simulink model "PDQuadrotor"  (Simulink 7.7)
settings: Solver=ode4  StartTime=0.0  StopTime=10.0  FixedStep=0.2  RelTol=1e-3
values from neighbouring files (symbols this model uses):
  b = 3.13*10^(-5)    (= 3.13e-05)    [Quadparameters.m]
  d = 7.5*10^(-7)    (= 7.5e-07)    [Quadparameters.m]
  g = 9.81    [Quadparameters.m]
  Ix = 7.5*10^(-3)    (= 0.0075)    [Quadparameters.m]
  Iy = 7.5*10^(-3)    (= 0.0075)    [Quadparameters.m]
  Iz = 1.3*10^(-2)    (= 0.013)    [Quadparameters.m]
  Jr = 6.5*10^(-5)    (= 6.5e-05)    [Quadparameters.m]
  kdp = 0.4    [Quadparameters.m]
  kdps = 0.4    [Quadparameters.m]
  kdt = 0.4    [Quadparameters.m]
  kdz = 20    [Quadparameters.m]
  kpp = 0.8    [Quadparameters.m]
  kpps = 1    [Quadparameters.m]
  kpt = 1.2    [Quadparameters.m]
  kpz = 100    [Quadparameters.m]
  l = 0.23    [Quadparameters.m]
  m = 0.65    [Quadparameters.m]
libraries: simulink x2
settings Model: Creator=abdelrazzak.merheb  LastModifiedBy=ISIT-Eric J.Huang
settings DebuggingCC: StrictBusMsg=Warning

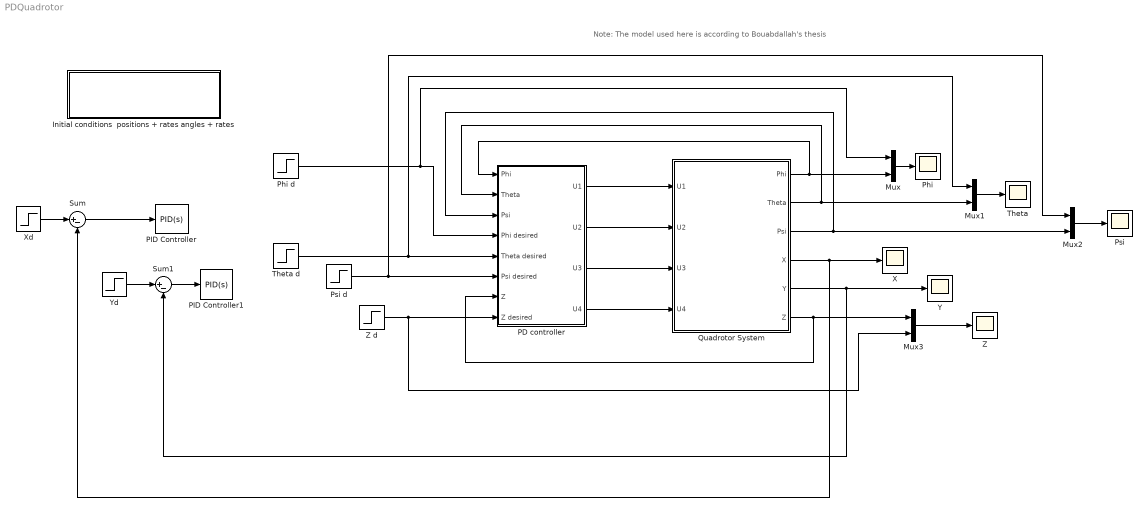
== system PDQuadrotor ==
  note: Note:
      | The model used here is according to Bouabdallah's thesis
  Initial conditions  positions + rates angles + rates : Subsystem  mask{x0=0, y0=0, z0=1, x0dot=0, y0dot=0, z0dot=0, phi0=0, theta0=0, psi0=0, phi0dot=0, theta0dot=0, psi0dot=0}
      mask prompts: x0 "Initial X position, in meters"; y0 "Initial Y position, in meters"; z0 "Initial Z position, in meters"; x0dot "Initial Velocity in X direction, m/sec"; y0dot "Initial Velocity in Y direction, m/sec"; z0dot "Initial Velocity in Z direction, m/sec"; phi0 "Initial Roll angle, deg"; theta0 "Initial Pitch angle, deg"; psi0 "Initial Yaw angle, deg"; phi0dot "Initial Roll rate, deg/sec"; theta0dot "Initial Pitch rate, deg/sec"; psi0dot "Initial Yaw rate, deg/sec"
      mask Display: disp('Enter initial conditions here')
  Mux{,1..3} (4 alike) : Mux  Inputs=2
  PD controller : Subsystem
  PID Controller : simulink/Continuous/PID Controller  SystemSampleTime=-1  Controller=PID  TimeDomain=Continuous-time  SampleTime=1  IntegratorMethod=Forward Euler  FilterMethod=Forward Euler  Form=Parallel  P=1  I=0  D=0  N=100  InitialConditionSource=internal  InitialConditionForIntegrator=0  InitialConditionForFilter=0  ExternalReset=none  LimitOutput=off  UpperSaturationLimit=inf  LowerSaturationLimit=-inf  LinearizeAsGain=off  AntiWindupMode=none  Kb=1  TrackingMode=off  Kt=1  PParamMin=[]  PParamMax=[]  IParamMin=[]  IParamMax=[]  DParamMin=[]  DParamMax=[]  NParamMin=[]  NParamMax=[]  KbParamMin=[]  KbParamMax=[]  KtParamMin=[]  KtParamMax=[]  POutMin=[]  POutMax=[]  IOutMin=[]  IOutMax=[]  DOutMin=[]  DOutMax=[]  NOutMin=[]  NOutMax=[]  KbOutMin=[]  KbOutMax=[]  KtOutMin=[]  KtOutMax=[]  IntegratorOutMin=[]  IntegratorOutMax=[]  FilterOutMin=[]  FilterOutMax=[]  SumOutMin=[]  SumOutMax=[]  SumI1OutMin=[]  SumI1OutMax=[]  SumI2OutMin=[]  SumI2OutMax=[]  SumI3OutMin=[]  SumI3OutMax=[]  SumDOutMin=[]  SumDOutMax=[]  SaturationOutMin=[]  SaturationOutMax=[]  IntegratorContinuousStateAttributes=''  IntegratorStateMustResolveToSignalObject=off  IntegratorRTWStateStorageClass=Auto  FilterContinuousStateAttributes=''  FilterStateMustResolveToSignalObject=off  FilterRTWStateStorageClass=Auto
  PID Controller1 : simulink/Continuous/PID Controller  SystemSampleTime=-1  Controller=PID  TimeDomain=Continuous-time  SampleTime=1  IntegratorMethod=Forward Euler  FilterMethod=Forward Euler  Form=Parallel  P=1  I=0  D=0  N=100  InitialConditionSource=internal  InitialConditionForIntegrator=0  InitialConditionForFilter=0  ExternalReset=none  LimitOutput=off  UpperSaturationLimit=inf  LowerSaturationLimit=-inf  LinearizeAsGain=off  AntiWindupMode=none  Kb=1  TrackingMode=off  Kt=1  PParamMin=[]  PParamMax=[]  IParamMin=[]  IParamMax=[]  DParamMin=[]  DParamMax=[]  NParamMin=[]  NParamMax=[]  KbParamMin=[]  KbParamMax=[]  KtParamMin=[]  KtParamMax=[]  POutMin=[]  POutMax=[]  IOutMin=[]  IOutMax=[]  DOutMin=[]  DOutMax=[]  NOutMin=[]  NOutMax=[]  KbOutMin=[]  KbOutMax=[]  KtOutMin=[]  KtOutMax=[]  IntegratorOutMin=[]  IntegratorOutMax=[]  FilterOutMin=[]  FilterOutMax=[]  SumOutMin=[]  SumOutMax=[]  SumI1OutMin=[]  SumI1OutMax=[]  SumI2OutMin=[]  SumI2OutMax=[]  SumI3OutMin=[]  SumI3OutMax=[]  SumDOutMin=[]  SumDOutMax=[]  SaturationOutMin=[]  SaturationOutMax=[]  IntegratorContinuousStateAttributes=''  IntegratorStateMustResolveToSignalObject=off  IntegratorRTWStateStorageClass=Auto  FilterContinuousStateAttributes=''  FilterStateMustResolveToSignalObject=off  FilterRTWStateStorageClass=Auto
  Phi : Scope
  Phi d : Step  After=0  SampleTime=0
  Psi : Scope
      settings: SaveName=ScopeData2
  Psi d : Step  After=0  SampleTime=0
  Quadrotor System : Subsystem
  Sum : Sum  Inputs=|+-
  Sum1 : Sum  Inputs=|+-
  Theta : Scope
  Theta d : Step  After=0.5  SampleTime=0
  X : Scope
      settings: SaveName=ScopeData3
  Xd : Step  Time=3  After=40  SampleTime=0
  Y : Scope
      settings: SaveName=ScopeData5
  Yd : Step  Time=5  After=35  SampleTime=0
  Z : Scope
      settings: SaveName=ScopeData4
  Z d : Step  Time=0  After=10  SampleTime=0
  wires:
  PD controller/1(U1) -> Quadrotor System/1(U1)
  PD controller/2(U2) -> Quadrotor System/2(U2)
  PD controller/3(U3) -> Quadrotor System/3(U3)
  PD controller/4(U4) -> Quadrotor System/4(U4)
  Quadrotor System/6(Z) -> PD controller/7(Z), Mux3/1
  Quadrotor System/1(Phi) -> PD controller/1(Phi), Mux/2
  Quadrotor System/2(Theta) -> PD controller/2(Theta), Mux1/2
  Quadrotor System/3(Psi) -> PD controller/3(Psi), Mux2/2
  Psi d/1 -> PD controller/6(Psi desired), Mux2/1
  Z d/1 -> PD controller/8(Z desired), Mux3/2
  Quadrotor System/5(Y) -> Y/1, Sum1/2
  Quadrotor System/4(X) -> X/1, Sum/2
  Mux/1 -> Phi/1
  Mux1/1 -> Theta/1
  Mux2/1 -> Psi/1
  Mux3/1 -> Z/1
  Sum1/1 -> PID Controller1/1
  Xd/1 -> Sum/1
  Sum/1 -> PID Controller/1
  Yd/1 -> Sum1/1
  Phi d/1 -> PD controller/4(Phi desired), Mux/1
  Theta d/1 -> PD controller/5(Theta desired), Mux1/1

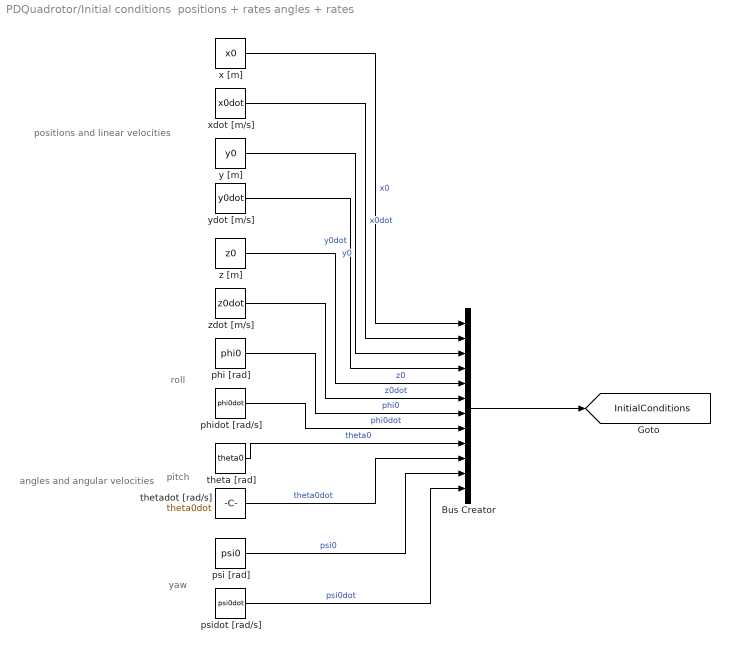
== system PDQuadrotor/Initial conditions  positions + rates angles + rates ==
  note: positions and linear velocities
  note: angles and angular velocities
  note: yaw
  note: pitch
  note: roll
  Bus Creator : BusCreator  Inputs=12
  phi [rad] : Constant  Value=phi0
  phidot [rad/s] : Constant  Value=phi0dot
  psi [rad] : Constant  Value=psi0
  psidot [rad/s] : Constant  Value=psi0dot
  theta [rad] : Constant  Value=theta0
  thetadot [rad/s] : Constant  Value=theta0dot
  x [m] : Constant  Value=x0
  xdot [m/s] : Constant  Value=x0dot
  y [m] : Constant  Value=y0
  ydot [m/s] : Constant  Value=y0dot
  z [m] : Constant  Value=z0
  zdot [m/s] : Constant  Value=z0dot
  tag scope: InitialConditions=global
  wires:
  x [m]/1 -> Bus Creator/1  "x0"
  xdot [m/s]/1 -> Bus Creator/2  "x0dot"
  y [m]/1 -> Bus Creator/3  "y0"
  ydot [m/s]/1 -> Bus Creator/4  "y0dot"
  z [m]/1 -> Bus Creator/5  "z0"
  zdot [m/s]/1 -> Bus Creator/6  "z0dot"
  phi [rad]/1 -> Bus Creator/7  "phi0"
  phidot [rad/s]/1 -> Bus Creator/8  "phi0dot"
  theta [rad]/1 -> Bus Creator/9  "theta0"
  thetadot [rad/s]/1 -> Bus Creator/10  "theta0dot"
  psi [rad]/1 -> Bus Creator/11  "psi0"
  psidot [rad/s]/1 -> Bus Creator/12  "psi0dot"
  Bus Creator/1 -> [InitialConditions]

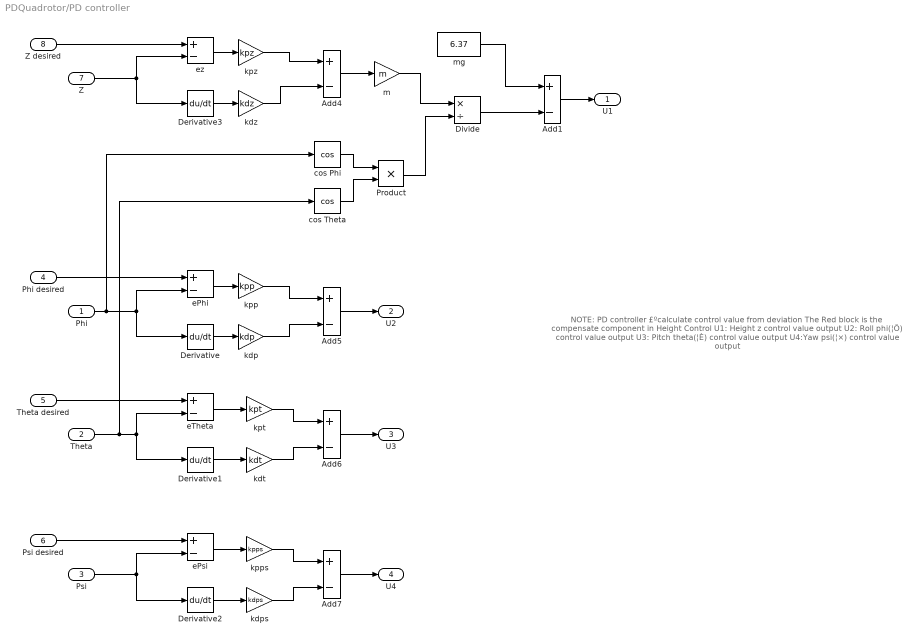
== system PDQuadrotor/PD controller ==
  note: NOTE:
      | PD controller £ºcalculate control value from deviation
      | The Red block is the compensate component in Height Control
      | U1: Height   z   control value output
      | U2: Roll  phi(¦Õ)  control value output
      | U3: Pitch  theta(¦È)  control value output
      | U4:Yaw  psi(¦×)  control value output
  Phi : Inport
  Theta : Inport  Port=2
  Psi : Inport  Port=3
  Phi desired : Inport  Port=4
  Theta desired : Inport  Port=5
  Psi desired : Inport  Port=6
  Z : Inport  Port=7
  Z desired : Inport  Port=8
  Add{1,4..7} (5 alike) : Sum  Inputs=+-
  Derivative{,1..3} (4 alike) : Derivative
  Divide : Product  Inputs=*/
  Product : Product  RndMeth=Zero
  cos Phi : Trigonometry  Operator=cos
  cos Theta : Trigonometry  Operator=cos
  ePhi : Sum  Inputs=+-
  ePsi : Sum  Inputs=+-
  eTheta : Sum  Inputs=+-
  ez : Sum  Inputs=+-
  kdp : Gain  Gain=kdp
  kdps : Gain  Gain=kdps
  kdt : Gain  Gain=kdt
  kdz : Gain  Gain=kdz
  kpp : Gain  Gain=kpp
  kpps : Gain  Gain=kpps
  kpt : Gain  Gain=kpt
  kpz : Gain  Gain=kpz
  m : Gain  Gain=m
  "mg " : Constant  Value=6.37
  U1 : Outport
  U2 : Outport  Port=2
  U3 : Outport  Port=3
  U4 : Outport  Port=4
  wires:
  Phi/1 -> Derivative/1, ePhi/2, cos Phi/1
  Theta/1 -> Derivative1/1, eTheta/2, cos Theta/1
  Psi/1 -> Derivative2/1, ePsi/2
  Phi desired/1 -> ePhi/1
  Theta desired/1 -> eTheta/1
  Psi desired/1 -> ePsi/1
  ePhi/1 -> kpp/1
  Derivative/1 -> kdp/1
  eTheta/1 -> kpt/1
  Derivative1/1 -> kdt/1
  ePsi/1 -> kpps/1
  Derivative2/1 -> kdps/1
  Z/1 -> Derivative3/1, ez/2
  Z desired/1 -> ez/1
  ez/1 -> kpz/1
  Derivative3/1 -> kdz/1
  kpz/1 -> Add4/1
  kdz/1 -> Add4/2
  kpp/1 -> Add5/1
  kdp/1 -> Add5/2
  Add5/1 -> U2/1
  kpt/1 -> Add6/1
  kdt/1 -> Add6/2
  Add6/1 -> U3/1
  kpps/1 -> Add7/1
  kdps/1 -> Add7/2
  Add7/1 -> U4/1
  cos Phi/1 -> Product/1
  cos Theta/1 -> Product/2
  Add4/1 -> m/1
  m/1 -> Divide/1
  Product/1 -> Divide/2
  "mg "/1 -> Add1/1
  Divide/1 -> Add1/2
  Add1/1 -> U1/1

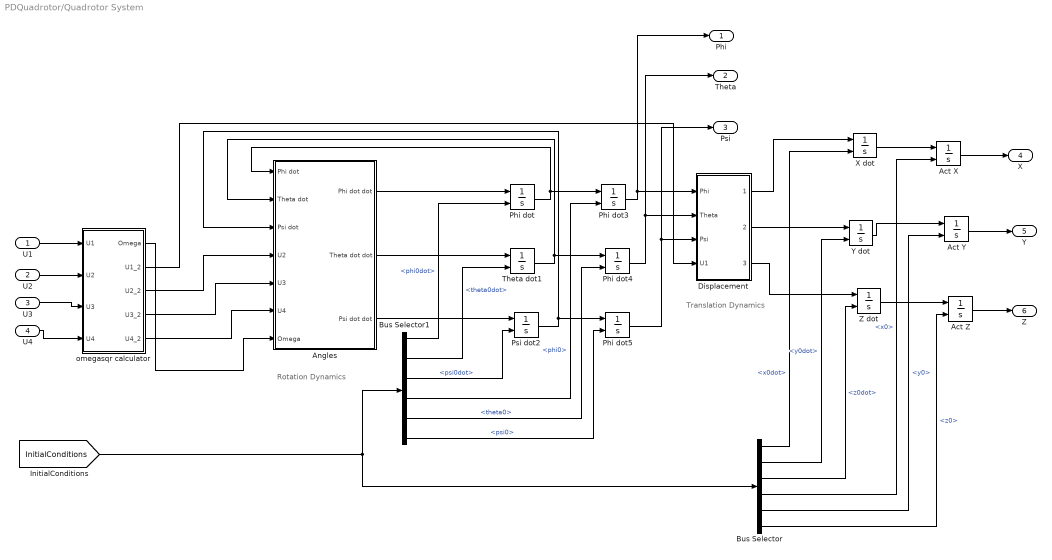
== system PDQuadrotor/Quadrotor System ==
  note: Rotation Dynamics
  note: Translation Dynamics
  U1 : Inport
  U2 : Inport  Port=2
  U3 : Inport  Port=3
  U4 : Inport  Port=4
  Act X : Integrator  InitialConditionSource=external
  Act Y : Integrator  InitialConditionSource=external
  Act Z : Integrator  InitialConditionSource=external
  Angles : Subsystem
  Bus Selector : BusSelector  OutputSignals=x0dot,y0dot,z0dot,x0,y0,z0
  Bus Selector1 : BusSelector  OutputSignals=phi0dot,theta0dot,psi0dot,phi0,theta0,psi0
  Displacement : Subsystem
  Phi dot : Integrator  InitialConditionSource=external
  Phi dot3 : Integrator  InitialConditionSource=external  ZeroCross=off
  Phi dot4 : Integrator  InitialConditionSource=external  ZeroCross=off
  Phi dot5 : Integrator  InitialConditionSource=external  ZeroCross=off
  Psi dot2 : Integrator  InitialConditionSource=external  ZeroCross=off
  Theta dot1 : Integrator  InitialConditionSource=external  ZeroCross=off
  X dot : Integrator  InitialConditionSource=external
  Y dot : Integrator  InitialConditionSource=external
  Z dot : Integrator  InitialConditionSource=external
  omegasqr calculator : Subsystem
  Phi : Outport
  Theta : Outport  Port=2
  Psi : Outport  Port=3
  X : Outport  Port=4
  Y : Outport  Port=5
  Z : Outport  Port=6
  wires:
  Angles/1(Phi dot dot) -> Phi dot/1
  Angles/2(Theta dot dot) -> Theta dot1/1
  Angles/3(Psi dot dot) -> Psi dot2/1
  Phi dot/1 -> Angles/1(Phi dot), Phi dot3/1
  Theta dot1/1 -> Angles/2(Theta dot), Phi dot4/1
  Psi dot2/1 -> Angles/3(Psi dot), Phi dot5/1
  omegasqr calculator/3(U2_2) -> Angles/4(U2)
  omegasqr calculator/4(U3_2) -> Angles/5(U3)
  omegasqr calculator/5(U4_2) -> Angles/6(U4)
  omegasqr calculator/1(Omega) -> Angles/7(Omega)
  Phi dot3/1 -> Displacement/1(Phi), Phi/1
  Phi dot4/1 -> Displacement/2(Theta), Theta/1
  Phi dot5/1 -> Displacement/3(Psi), Psi/1
  omegasqr calculator/2(U1_2) -> Displacement/4(U1)
  Displacement/1(x dotdot) -> X dot/1
  X dot/1 -> Act X/1
  Y dot/1 -> Act Y/1
  Displacement/2(y dotdot) -> Y dot/1
  Z dot/1 -> Act Z/1
  Displacement/3(z dotdot) -> Z dot/1
  Act X/1 -> X/1
  Act Y/1 -> Y/1
  Act Z/1 -> Z/1
  U1/1 -> omegasqr calculator/1(U1)
  U2/1 -> omegasqr calculator/2(U2)
  U3/1 -> omegasqr calculator/3(U3)
  U4/1 -> omegasqr calculator/4(U4)
  [InitialConditions] -> Bus Selector/1, Bus Selector1/1
  Bus Selector1/1 -> Phi dot/2  "<phi0dot>"
  Bus Selector1/2 -> Theta dot1/2  "<theta0dot>"
  Bus Selector1/3 -> Psi dot2/2  "<psi0dot>"
  Bus Selector1/4 -> Phi dot3/2  "<phi0>"
  Bus Selector1/5 -> Phi dot4/2  "<theta0>"
  Bus Selector1/6 -> Phi dot5/2  "<psi0>"
  Bus Selector/1 -> X dot/2  "<x0dot>"
  Bus Selector/2 -> Y dot/2  "<y0dot>"
  Bus Selector/3 -> Z dot/2  "<z0dot>"
  Bus Selector/4 -> Act X/2  "<x0>"
  Bus Selector/5 -> Act Y/2  "<y0>"
  Bus Selector/6 -> Act Z/2  "<z0>"

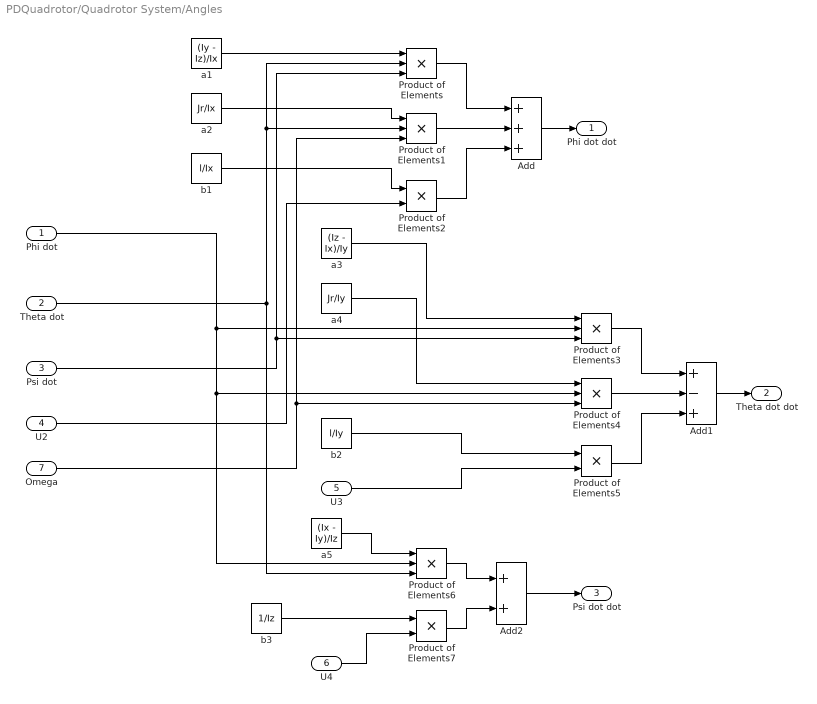
== system PDQuadrotor/Quadrotor System/Angles ==
  Phi dot : Inport
  Theta dot : Inport  Port=2
  Psi dot : Inport  Port=3
  U2 : Inport  Port=4
  U3 : Inport  Port=5
  U4 : Inport  Port=6
  Omega : Inport  Port=7
  Add : Sum  Inputs=+++
  Add1 : Sum  Inputs=+-+
  Add2 : Sum
  Product of Elements{,1,3..4,6} (5 alike) : Product  Inputs=3
  Product of Elements2 : Product
  Product of Elements5 : Product
  Product of Elements7 : Product
  a1 : Constant  Value=(Iy - Iz)/Ix
  a2 : Constant  Value=Jr/Ix
  a3 : Constant  Value=(Iz - Ix)/Iy
  a4 : Constant  Value=Jr/Iy
  a5 : Constant  Value=(Ix - Iy)/Iz
  b1 : Constant  Value=l/Ix
  b2 : Constant  Value=l/Iy
  b3 : Constant  Value=1/Iz
  Phi dot dot : Outport
  Theta dot dot : Outport  Port=2
  Psi dot dot : Outport  Port=3
  wires:
  Product of Elements/1 -> Add/1
  Product of Elements1/1 -> Add/2
  Product of Elements2/1 -> Add/3
  Add/1 -> Phi dot dot/1
  a1/1 -> Product of Elements/1
  Theta dot/1 -> Product of Elements/2, Product of Elements1/2, Product of Elements6/3
  Psi dot/1 -> Product of Elements/3, Product of Elements3/3
  a2/1 -> Product of Elements1/1
  b1/1 -> Product of Elements2/1
  U2/1 -> Product of Elements2/2
  Omega/1 -> Product of Elements1/3, Product of Elements4/3
  Product of Elements3/1 -> Add1/1
  Product of Elements4/1 -> Add1/2
  Product of Elements5/1 -> Add1/3
  Add1/1 -> Theta dot dot/1
  a3/1 -> Product of Elements3/1
  a4/1 -> Product of Elements4/1
  b2/1 -> Product of Elements5/1
  U3/1 -> Product of Elements5/2
  Phi dot/1 -> Product of Elements3/2, Product of Elements4/2, Product of Elements6/2
  Product of Elements6/1 -> Add2/1
  Product of Elements7/1 -> Add2/2
  Add2/1 -> Psi dot dot/1
  U4/1 -> Product of Elements7/2
  b3/1 -> Product of Elements7/1
  a5/1 -> Product of Elements6/1

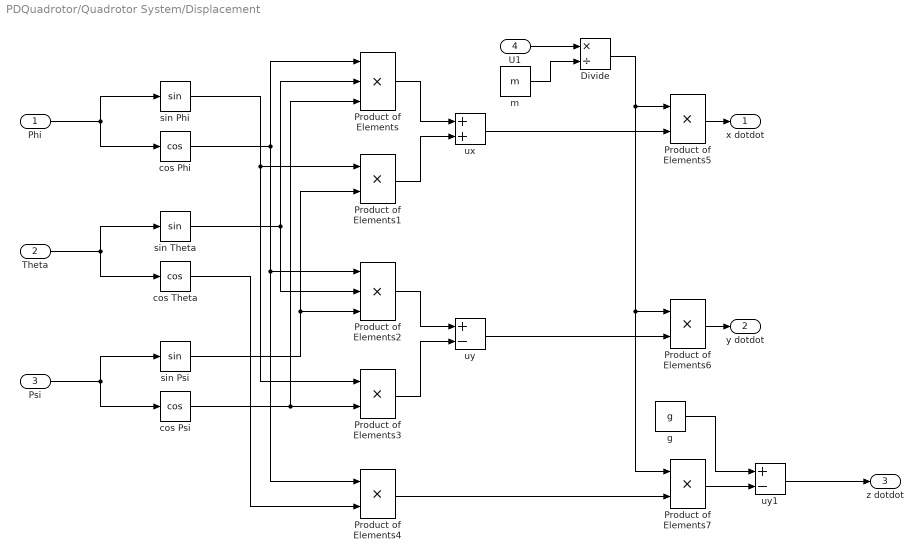
== system PDQuadrotor/Quadrotor System/Displacement ==
  Phi : Inport
  Theta : Inport  Port=2
  Psi : Inport  Port=3
  U1 : Inport  Port=4
  Divide : Product  Inputs=*/
  Product of Elements : Product  Inputs=3
  Product of Elements{1,3..7} (6 alike) : Product
  Product of Elements2 : Product  Inputs=3
  cos Phi : Trigonometry  Operator=cos
  cos Psi : Trigonometry  Operator=cos
  cos Theta : Trigonometry  Operator=cos
  g : Constant  Value=g
  m : Constant  Value=m
  sin Phi : Trigonometry
  sin Psi : Trigonometry
  sin Theta : Trigonometry
  ux : Sum
  uy : Sum  Inputs=+-
  uy1 : Sum  Inputs=+-
  x dotdot : Outport
  y dotdot : Outport  Port=2
  z dotdot : Outport  Port=3
  wires:
  Phi/1 -> sin Phi/1, cos Phi/1
  Theta/1 -> sin Theta/1, cos Theta/1
  Psi/1 -> sin Psi/1, cos Psi/1
  sin Theta/1 -> Product of Elements/2, Product of Elements2/2
  cos Psi/1 -> Product of Elements/3, Product of Elements3/2
  cos Phi/1 -> Product of Elements/1, Product of Elements2/1, Product of Elements4/1
  sin Phi/1 -> Product of Elements1/1, Product of Elements3/1
  sin Psi/1 -> Product of Elements1/2, Product of Elements2/3
  Product of Elements/1 -> ux/1
  Product of Elements1/1 -> ux/2
  ux/1 -> Product of Elements5/2
  Product of Elements2/1 -> uy/1
  Product of Elements3/1 -> uy/2
  uy/1 -> Product of Elements6/2
  cos Theta/1 -> Product of Elements4/2
  Product of Elements4/1 -> Product of Elements7/2
  U1/1 -> Divide/1
  m/1 -> Divide/2
  Divide/1 -> Product of Elements5/1, Product of Elements6/1, Product of Elements7/1
  Product of Elements5/1 -> x dotdot/1
  Product of Elements6/1 -> y dotdot/1
  uy1/1 -> z dotdot/1
  Product of Elements7/1 -> uy1/2
  g/1 -> uy1/1

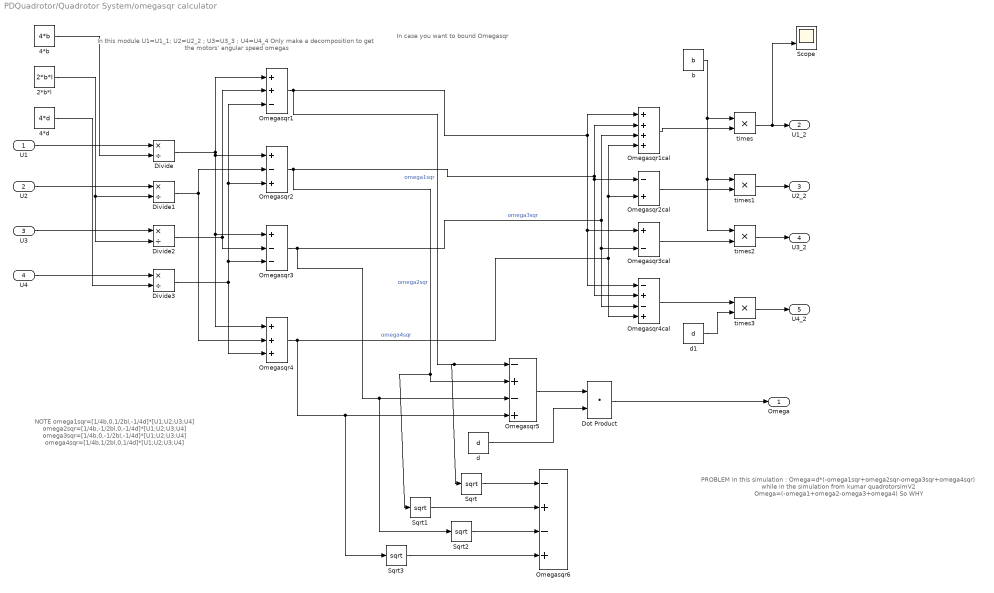
== system PDQuadrotor/Quadrotor System/omegasqr calculator ==
  note: In case you want to bound Omegasqr
  note: NOTE
      | omega1sqr=[1/4b,0,1/2bl,-1/4d]*[U1;U2;U3;U4]
      | omega2sqr=[1/4b,-1/2bl,0,-1/4d]*[U1;U2;U3;U4]
      | omega3sqr=[1/4b,0,-1/2bl,-1/4d]*[U1;U2;U3;U4]
      | omega4sqr=[1/4b,1/2bl,0,1/4d]*[U1;U2;U3;U4]
  note: PROBLEM
      | In this simulation :
      | Omega=d*(-omega1sqr+omega2sqr-omega3sqr+omega4sqr)
      | while in the simulation from kumar quadrotorsimV2
      | Omega=(-omega1+omega2-omega3+omega4)
      | So WHY
  note: In this module
      | U1=U1_1;  U2=U2_2 ; U3=U3_3 ; U4=U4_4
      | Only make a decomposition to get the motors' angular speed omegas
  U1 : Inport
  U2 : Inport  Port=2
  U3 : Inport  Port=3
  U4 : Inport  Port=4
  2*b*l : Constant  Value=2*b*l
  4*b : Constant  Value=4*b
  4*d : Constant  Value=4*d
  Divide{,1..3} (4 alike) : Product  Inputs=*/
  Dot Product : DotProduct  InputSameDT=on  OutDataTypeStr=Inherit: Inherit via internal rule
  Omegasqr1 : Sum  Inputs=++-
  Omegasqr1cal : Sum  Inputs=++++
  Omegasqr2 : Sum  Inputs=+-+
  Omegasqr2cal : Sum  Inputs=-+
  Omegasqr3 : Sum  Inputs=+--
  Omegasqr3cal : Sum  Inputs=+-
  Omegasqr4 : Sum  Inputs=+++
  Omegasqr4cal : Sum  Inputs=-+-+
  Omegasqr5 : Sum  Inputs=-+-+
  Omegasqr6 : Sum  Inputs=-+-+
  Scope : Scope  NumInputPorts=2
      settings: YMin=-5~-5  YMax=5~5  SaveName=ScopeData6
  Sqrt{,1..3} (4 alike) : Sqrt  SaturateOnIntegerOverflow=on
  b : Constant  Value=b
  d : Constant  Value=d
  d1 : Constant  Value=d
  times{,1..3} (4 alike) : Product  Inputs=**
  Omega : Outport
  U1_2 : Outport  Port=2
  U2_2 : Outport  Port=3
  U3_2 : Outport  Port=4
  U4_2 : Outport  Port=5
  wires:
  U1/1 -> Divide/1
  4*b/1 -> Divide/2
  U2/1 -> Divide1/1
  2*b*l/1 -> Divide1/2, Divide2/2
  U3/1 -> Divide2/1
  U4/1 -> Divide3/1
  4*d/1 -> Divide3/2
  Divide/1 -> Omegasqr1/1, Omegasqr2/1, Omegasqr3/1, Omegasqr4/1
  Divide2/1 -> Omegasqr1/2, Omegasqr3/2
  Divide3/1 -> Omegasqr1/3, Omegasqr2/3, Omegasqr3/3, Omegasqr4/3
  Divide1/1 -> Omegasqr2/2, Omegasqr4/2
  Omegasqr1/1 -> Omegasqr1cal/1, Omegasqr3cal/1, Omegasqr4cal/1, Omegasqr5/1, Sqrt/1  "omega1sqr"
  Omegasqr2/1 -> Omegasqr1cal/2, Omegasqr2cal/1, Omegasqr4cal/2, Omegasqr5/2, Sqrt1/1  "omega2sqr"
  Omegasqr3/1 -> Omegasqr1cal/3, Omegasqr3cal/2, Omegasqr4cal/3, Omegasqr5/3, Sqrt2/1  "omega3sqr"
  Omegasqr4/1 -> Omegasqr1cal/4, Omegasqr2cal/2, Omegasqr4cal/4, Omegasqr5/4, Sqrt3/1  "omega4sqr"
  Omegasqr5/1 -> Dot Product/1
  d/1 -> Dot Product/2
  b/1 -> times/1, times1/1, times2/1
  Omegasqr1cal/1 -> times/2
  Omegasqr2cal/1 -> times1/2
  Omegasqr3cal/1 -> times2/2
  Omegasqr4cal/1 -> times3/1
  d1/1 -> times3/2
  times/1 -> U1_2/1, Scope/2
  times1/1 -> U2_2/1
  times3/1 -> U4_2/1
  times2/1 -> U3_2/1
  Sqrt/1 -> Omegasqr6/1
  Sqrt1/1 -> Omegasqr6/2
  Sqrt2/1 -> Omegasqr6/3
  Sqrt3/1 -> Omegasqr6/4
  Dot Product/1 -> Omega/1
